simulink model "MATLABPSB_BASED_MODELING_AND_Sim"  (Simulink 8.1)
settings: Solver=FixedStepDiscrete  SolverMode=SingleTasking  StartTime=0.0  StopTime=1  FixedStep=Ts  MaxStep=Ts*2  RelTol=1e-4  AbsTol=1e-4
PreLoadFcn:
  | Ts=50e-6;
values from neighbouring files (symbols this model uses):
  A = 1.5    [LoadSimulation.m]
undefined symbols (not defined in the file or in its folder): DiscIntNeverNeededParam, find_system
libraries: powerlib x205, powerlib_extras x39
(part 2 of 5)

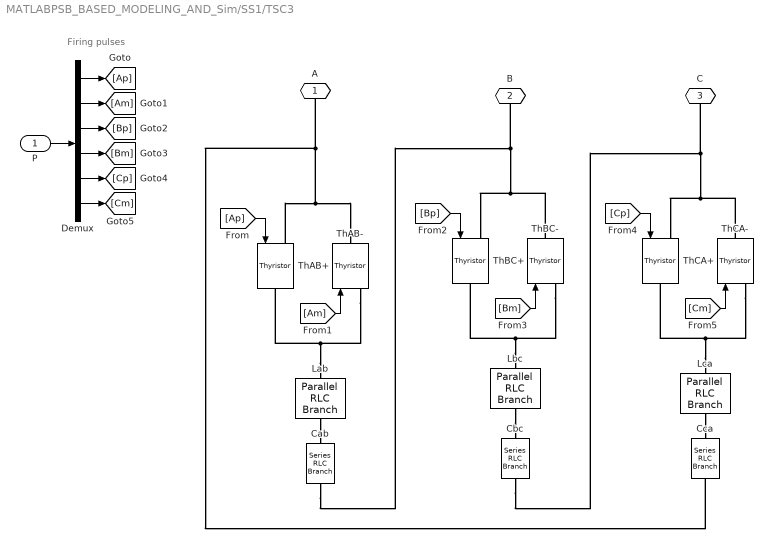
== system MATLABPSB_BASED_MODELING_AND_Sim/SS1/TSC3 ==
  note: Firing pulses
  P : Inport  PortDimensions=6
  Cab : powerlib/Elements/Series RLC Branch  LConnTagsString=__new0  RConnTagsString=__new0  BranchType=RC  Resistance=Rseries  Inductance=1.0  SetiL0=off  InitialCurrent=0  Capacitance=Ccmt  Setx0=off  InitialVoltage=0  Measurements=Branch voltage and current
  Cbc : powerlib/Elements/Series RLC Branch  LConnTagsString=__new0  RConnTagsString=__new0  BranchType=RC  Resistance=Rseries  Inductance=1.0  SetiL0=off  InitialCurrent=0  Capacitance=Ccmt  Setx0=off  InitialVoltage=0  Measurements=None
  Cca : powerlib/Elements/Series RLC Branch  LConnTagsString=__new0  RConnTagsString=__new0  BranchType=RC  Resistance=Rseries  Inductance=1.0  SetiL0=off  InitialCurrent=0  Capacitance=Ccmt  Setx0=off  InitialVoltage=0  Measurements=None
  Demux : Demux  Outputs=6
  Lab : powerlib/Elements/Parallel RLC Branch  LConnTagsString=a  RConnTagsString=__new0  BranchType=RL  Resistance=Rparallel  Inductance=Lcmt  SetiL0=off  InitialCurrent=0  Capacitance=1.0  Setx0=off  InitialVoltage=0  Measurements=None
  Lbc : powerlib/Elements/Parallel RLC Branch  LConnTagsString=a  RConnTagsString=__new0  BranchType=RL  Resistance=Rparallel  Inductance=Lcmt  SetiL0=off  InitialCurrent=0  Capacitance=1.0  Setx0=off  InitialVoltage=0  Measurements=None
  Lca : powerlib/Elements/Parallel RLC Branch  LConnTagsString=a  RConnTagsString=__new0  BranchType=RL  Resistance=Rparallel  Inductance=Lcmt  SetiL0=off  InitialCurrent=0  Capacitance=1.0  Setx0=off  InitialVoltage=0  Measurements=None
  ThAB+ : powerlib/Power Electronics/Thyristor  Ron=Ron  Lon=0  Vf=Vf  IC=0  Rs=Rsnub  Cs=Csnub  Measurements=off
      settings: AttributesFormatString=\n
  ThAB- : powerlib/Power Electronics/Thyristor  Ron=Ron  Lon=0  Vf=Vf  IC=0  Rs=inf  Cs=0  Measurements=off
      settings: AttributesFormatString=\n
  ThBC+ : powerlib/Power Electronics/Thyristor  Ron=Ron  Lon=0  Vf=Vf  IC=0  Rs=Rsnub  Cs=Csnub  Measurements=off
      settings: AttributesFormatString=\n
  ThBC- : powerlib/Power Electronics/Thyristor  Ron=Ron  Lon=0  Vf=Vf  IC=0  Rs=inf  Cs=0  Measurements=off
      settings: AttributesFormatString=\n
  ThCA+ : powerlib/Power Electronics/Thyristor  Ron=Ron  Lon=0  Vf=Vf  IC=0  Rs=Rsnub  Cs=Csnub  Measurements=off
      settings: AttributesFormatString=\n
  ThCA- : powerlib/Power Electronics/Thyristor  Ron=Ron  Lon=0  Vf=Vf  IC=0  Rs=inf  Cs=0  Measurements=off
      settings: AttributesFormatString=\n
  A : PMIOPort  Port=1  Side=Left
  B : PMIOPort  Port=2  Side=Left
  C : PMIOPort  Port=3  Side=Left
  wires:
  P/1 -> Demux/1
  [Ap] -> ThAB+/1
  Demux/1 -> [Ap]
  Demux/2 -> [Am]
  Demux/3 -> [Bp]
  Demux/4 -> [Bm]
  Demux/5 -> [Cp]
  [Am] -> ThAB-/1
  [Bp] -> ThBC+/1
  [Bm] -> ThBC-/1
  [Cp] -> ThCA+/1
  [Cm] -> ThCA-/1
  Demux/6 -> [Cm]
  connections:
  Lab/RConn1 -- Cab/LConn1
  Lab/LConn1 -- ThAB-/LConn1 -- ThAB+/RConn1
  Cca/RConn1 -- A/RConn1 -- ThAB+/LConn1 -- ThAB-/RConn1
  Lbc/LConn1 -- ThBC-/LConn1 -- ThBC+/RConn1
  Cab/RConn1 -- ThBC-/RConn1 -- ThBC+/LConn1 -- B/RConn1
  Lca/LConn1 -- ThCA-/LConn1 -- ThCA+/RConn1
  Cbc/RConn1 -- ThCA-/RConn1 -- ThCA+/LConn1 -- C/RConn1
  Lbc/RConn1 -- Cbc/LConn1
  Lca/RConn1 -- Cca/LConn1

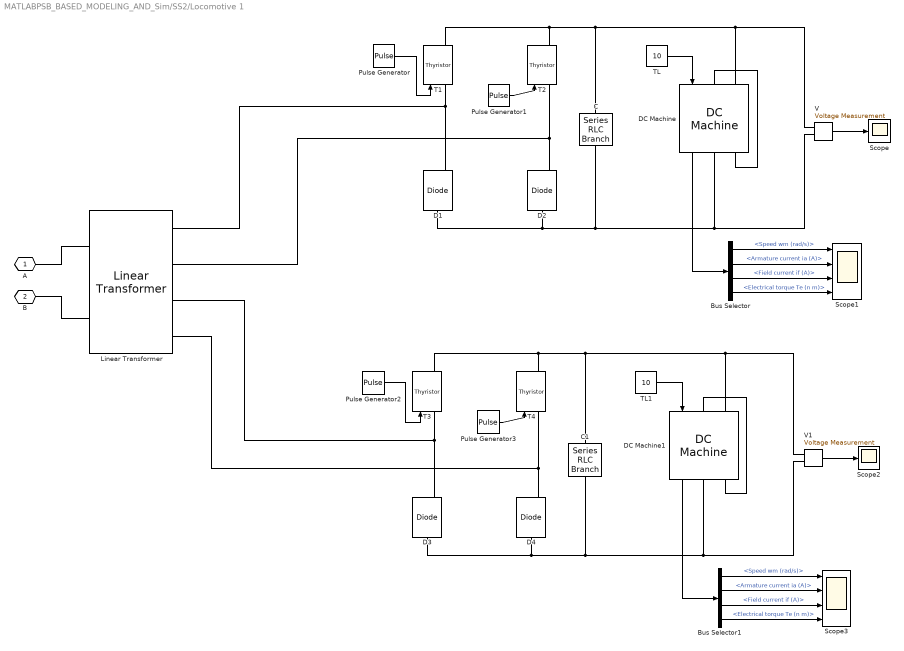
== system MATLABPSB_BASED_MODELING_AND_Sim/SS2/Locomotive 1 ==
  Bus Selector : BusSelector  OutputSignals=Speed wm (rad/s),Armature current ia (A),Field current if (A),Electrical torque Te (n m)
  Bus Selector1 : BusSelector  OutputSignals=Speed wm (rad/s),Armature current ia (A),Field current if (A),Electrical torque Te (n m)
  C : powerlib/Elements/Series RLC Branch  LConnTagsString=__new0  RConnTagsString=__new0  BranchType=C  Resistance=1000  Inductance=1e-3  SetiL0=off  InitialCurrent=0  Capacitance=2000e-6  Setx0=on  InitialVoltage=400  Measurements=None
  C1 : powerlib/Elements/Series RLC Branch  LConnTagsString=__new0  RConnTagsString=__new0  BranchType=C  Resistance=1000  Inductance=1e-3  SetiL0=off  InitialCurrent=0  Capacitance=2000e-6  Setx0=on  InitialVoltage=400  Measurements=None
  D{1..4} (4 alike) : powerlib/Power Electronics/Diode  Ron=0.001  Lon=0  Vf=0.8  IC=0  UseSnubber=off  Rs=500  Cs=250e-9  Measurements=on
  DC Machine : powerlib/Machines/DC Machine  PresetModel=No  MechanicalLoad=Torque TL  FieldType=Wound  ShowDetailedParameters=on  RLa="[ 2.6  150e-3]"  RLf=[0.6 20e-3]  Laf=1.8  MachineConstant=Torque constant (N.m/A)  Ke=1.8  Kt=1.8  J=0.1  Bm=0  Tf=0  w0=1  Ifinit=1  TsPowergui=0  TsBlock=-1
  DC Machine1 : powerlib/Machines/DC Machine  PresetModel=No  MechanicalLoad=Torque TL  FieldType=Wound  ShowDetailedParameters=on  RLa="[ 2.6  150e-3]"  RLf=[0.6 20e-3]  Laf=1.8  MachineConstant=Torque constant (N.m/A)  Ke=1.8  Kt=1.8  J=0.1  Bm=0  Tf=0  w0=1  Ifinit=1  TsPowergui=0  TsBlock=-1
  Linear Transformer : powerlib/Elements/Linear Transformer  LConnTagsString=a|b  RConnTagsString=A|B|C|D  UNITS=pu  NominalPower=[ 10e6 50 ]  winding1="[ 25e3  0.0001  0.04 ]"  winding2="[ 400  0.0001  0.02 ]"  ThreeWindings=on  winding3="[ 400  0.0001  0.02 ]"  RmLm=[ 500 500 ]  Measurements=None  DataType=off
  Pulse Generator : DiscretePulseGenerator  PulseType=Time based  Period=20e-3  PulseWidth=3
  Pulse Generator1 : DiscretePulseGenerator  PulseType=Time based  Period=20e-3  PulseWidth=3  PhaseDelay=10e-3
  Pulse Generator2 : DiscretePulseGenerator  PulseType=Time based  Period=20e-3  PulseWidth=3
  Pulse Generator3 : DiscretePulseGenerator  PulseType=Time based  Period=20e-3  PulseWidth=3  PhaseDelay=10e-3
  Scope : Scope
      settings: YMin=-50  YMax=800  SaveName=ScopeData3  Decimation=5
  Scope1 : Scope  NumInputPorts=4
      settings: YMin=0~-5~-5~-5  YMax=100~5~5~20  SaveName=ScopeData4  Decimation=5
  Scope2 : Scope
      settings: YMin=-50  YMax=800  SaveName=ScopeData5  Decimation=5
  Scope3 : Scope  NumInputPorts=4
      settings: YMin=0~-5~-5~-5  YMax=100~5~5~20  SaveName=ScopeData6  Decimation=5
  T{1..4} (4 alike) : powerlib/Power Electronics/Thyristor  Ron=0.001  Lon=0  Vf=0.8  IC=0  Rs=500  Cs=250e-9  Measurements=on
  TL : Constant  Value=10
  TL1 : Constant  Value=10
  V : powerlib/Measurements/Voltage Measurement  PhasorSimulation=off  OutputType=Complex  PSBequivalent=0
  V1 : powerlib/Measurements/Voltage Measurement  PhasorSimulation=off  OutputType=Complex  PSBequivalent=0
  A : PMIOPort  Tag=PMCPort  Port=1  Side=Left
  B : PMIOPort  Tag=PMCPort  Port=2  Side=Left
  wires:
  Pulse Generator/1 -> T1/1
  Pulse Generator1/1 -> T2/1
  V/1 -> Scope/1
  TL/1 -> DC Machine/1
  DC Machine/1 -> Bus Selector/1
  Bus Selector/1 -> Scope1/1  "<Speed wm (rad/s)>"
  Bus Selector/2 -> Scope1/2  "<Armature current ia (A)>"
  Bus Selector/3 -> Scope1/3  "<Field current if (A)>"
  Bus Selector/4 -> Scope1/4  "<Electrical torque Te (n m)>"
  Pulse Generator2/1 -> T3/1
  Pulse Generator3/1 -> T4/1
  V1/1 -> Scope2/1
  TL1/1 -> DC Machine1/1
  DC Machine1/1 -> Bus Selector1/1
  Bus Selector1/1 -> Scope3/1  "<Speed wm (rad/s)>"
  Bus Selector1/2 -> Scope3/2  "<Armature current ia (A)>"
  Bus Selector1/3 -> Scope3/3  "<Field current if (A)>"
  Bus Selector1/4 -> Scope3/4  "<Electrical torque Te (n m)>"
  connections:
  D1/RConn1 -- Linear Transformer/RConn1 -- T1/LConn1
  D2/RConn1 -- Linear Transformer/RConn2 -- T2/LConn1
  T1/RConn1 -- T2/RConn1 -- C/LConn1 -- V/LConn1 -- DC Machine/LConn2
  D1/LConn1 -- D2/LConn1 -- C/RConn1 -- V/LConn2 -- DC Machine/RConn1
  DC Machine/RConn2 -- DC Machine/LConn1
  T3/RConn1 -- T4/RConn1 -- V1/LConn1 -- DC Machine1/LConn2 -- C1/LConn1
  D3/LConn1 -- D4/LConn1 -- V1/LConn2 -- DC Machine1/RConn1 -- C1/RConn1
  DC Machine1/RConn2 -- DC Machine1/LConn1
  D4/RConn1 -- T4/LConn1 -- Linear Transformer/RConn4
  D3/RConn1 -- T3/LConn1 -- Linear Transformer/RConn3
  A/RConn1 -- Linear Transformer/LConn1
  B/RConn1 -- Linear Transformer/LConn2

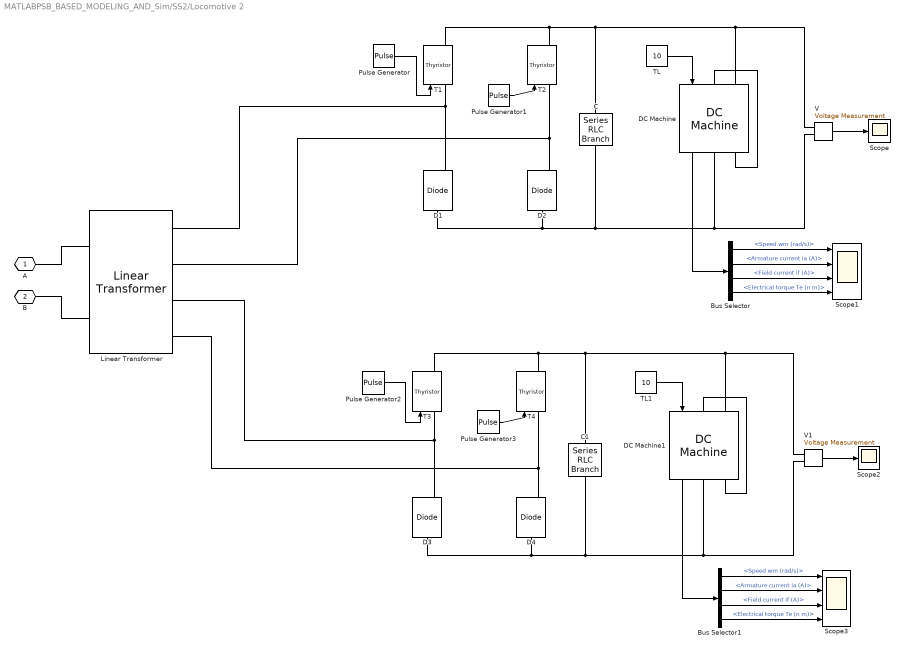
== system MATLABPSB_BASED_MODELING_AND_Sim/SS2/Locomotive 2 ==
  Bus Selector : BusSelector  OutputSignals=Speed wm (rad/s),Armature current ia (A),Field current if (A),Electrical torque Te (n m)
  Bus Selector1 : BusSelector  OutputSignals=Speed wm (rad/s),Armature current ia (A),Field current if (A),Electrical torque Te (n m)
  C : powerlib/Elements/Series RLC Branch  LConnTagsString=__new0  RConnTagsString=__new0  BranchType=C  Resistance=1000  Inductance=1e-3  SetiL0=off  InitialCurrent=0  Capacitance=2000e-6  Setx0=on  InitialVoltage=400  Measurements=None
  C1 : powerlib/Elements/Series RLC Branch  LConnTagsString=__new0  RConnTagsString=__new0  BranchType=C  Resistance=1000  Inductance=1e-3  SetiL0=off  InitialCurrent=0  Capacitance=2000e-6  Setx0=on  InitialVoltage=400  Measurements=None
  D{1..4} (4 alike) : powerlib/Power Electronics/Diode  Ron=0.001  Lon=0  Vf=0.8  IC=0  UseSnubber=off  Rs=500  Cs=250e-9  Measurements=on
  DC Machine : powerlib/Machines/DC Machine  PresetModel=No  MechanicalLoad=Torque TL  FieldType=Wound  ShowDetailedParameters=on  RLa="[ 2.6  150e-3]"  RLf=[0.6 20e-3]  Laf=1.8  MachineConstant=Torque constant (N.m/A)  Ke=1.8  Kt=1.8  J=0.1  Bm=0  Tf=0  w0=1  Ifinit=1  TsPowergui=0  TsBlock=-1
  DC Machine1 : powerlib/Machines/DC Machine  PresetModel=No  MechanicalLoad=Torque TL  FieldType=Wound  ShowDetailedParameters=on  RLa="[ 2.6  150e-3]"  RLf=[0.6 20e-3]  Laf=1.8  MachineConstant=Torque constant (N.m/A)  Ke=1.8  Kt=1.8  J=0.1  Bm=0  Tf=0  w0=1  Ifinit=1  TsPowergui=0  TsBlock=-1
  Linear Transformer : powerlib/Elements/Linear Transformer  LConnTagsString=a|b  RConnTagsString=A|B|C|D  UNITS=pu  NominalPower=[ 10e6 50 ]  winding1="[ 25e3  0.0001  0.04 ]"  winding2="[ 400  0.0001  0.02 ]"  ThreeWindings=on  winding3="[ 400  0.0001  0.02 ]"  RmLm=[ 500 500 ]  Measurements=None  DataType=off
  Pulse Generator : DiscretePulseGenerator  PulseType=Time based  Period=20e-3  PulseWidth=3
  Pulse Generator1 : DiscretePulseGenerator  PulseType=Time based  Period=20e-3  PulseWidth=3  PhaseDelay=10e-3
  Pulse Generator2 : DiscretePulseGenerator  PulseType=Time based  Period=20e-3  PulseWidth=3
  Pulse Generator3 : DiscretePulseGenerator  PulseType=Time based  Period=20e-3  PulseWidth=3  PhaseDelay=10e-3
  Scope : Scope
      settings: YMin=-50  YMax=800  SaveName=ScopeData3  Decimation=5
  Scope1 : Scope  NumInputPorts=4
      settings: YMin=0~-5~-5~-5  YMax=100~5~5~20  SaveName=ScopeData4  Decimation=5
  Scope2 : Scope
      settings: YMin=-50  YMax=800  SaveName=ScopeData5  Decimation=5
  Scope3 : Scope  NumInputPorts=4
      settings: YMin=0~-5~-5~-5  YMax=100~5~5~20  SaveName=ScopeData6  Decimation=5
  T{1..4} (4 alike) : powerlib/Power Electronics/Thyristor  Ron=0.001  Lon=0  Vf=0.8  IC=0  Rs=500  Cs=250e-9  Measurements=on
  TL : Constant  Value=10
  TL1 : Constant  Value=10
  V : powerlib/Measurements/Voltage Measurement  PhasorSimulation=off  OutputType=Complex  PSBequivalent=0
  V1 : powerlib/Measurements/Voltage Measurement  PhasorSimulation=off  OutputType=Complex  PSBequivalent=0
  A : PMIOPort  Tag=PMCPort  Port=1  Side=Left
  B : PMIOPort  Tag=PMCPort  Port=2  Side=Left
  wires:
  Pulse Generator/1 -> T1/1
  Pulse Generator1/1 -> T2/1
  V/1 -> Scope/1
  TL/1 -> DC Machine/1
  DC Machine/1 -> Bus Selector/1
  Bus Selector/1 -> Scope1/1  "<Speed wm (rad/s)>"
  Bus Selector/2 -> Scope1/2  "<Armature current ia (A)>"
  Bus Selector/3 -> Scope1/3  "<Field current if (A)>"
  Bus Selector/4 -> Scope1/4  "<Electrical torque Te (n m)>"
  Pulse Generator2/1 -> T3/1
  Pulse Generator3/1 -> T4/1
  V1/1 -> Scope2/1
  TL1/1 -> DC Machine1/1
  DC Machine1/1 -> Bus Selector1/1
  Bus Selector1/1 -> Scope3/1  "<Speed wm (rad/s)>"
  Bus Selector1/2 -> Scope3/2  "<Armature current ia (A)>"
  Bus Selector1/3 -> Scope3/3  "<Field current if (A)>"
  Bus Selector1/4 -> Scope3/4  "<Electrical torque Te (n m)>"
  connections:
  D1/RConn1 -- Linear Transformer/RConn1 -- T1/LConn1
  D2/RConn1 -- Linear Transformer/RConn2 -- T2/LConn1
  T1/RConn1 -- T2/RConn1 -- C/LConn1 -- V/LConn1 -- DC Machine/LConn2
  D1/LConn1 -- D2/LConn1 -- C/RConn1 -- V/LConn2 -- DC Machine/RConn1
  DC Machine/RConn2 -- DC Machine/LConn1
  T3/RConn1 -- T4/RConn1 -- V1/LConn1 -- DC Machine1/LConn2 -- C1/LConn1
  D3/LConn1 -- D4/LConn1 -- V1/LConn2 -- DC Machine1/RConn1 -- C1/RConn1
  DC Machine1/RConn2 -- DC Machine1/LConn1
  D4/RConn1 -- T4/LConn1 -- Linear Transformer/RConn4
  D3/RConn1 -- T3/LConn1 -- Linear Transformer/RConn3
  A/RConn1 -- Linear Transformer/LConn1
  B/RConn1 -- Linear Transformer/LConn2

== system MATLABPSB_BASED_MODELING_AND_Sim/SS2/SVC Controller ==
  note: Pulses
  note: SVC Controller
  note: Pierre Giroux, Gilbert Sybille
      | Power System Laboratory, IREQ
      | Hydro-Quebec
  note: used for misfiring
      | simulation
  Vabc_prim : Inport  PortDimensions=3
  Vabc_sec : Inport  Port=2  PortDimensions=3
  3-phase signal generator : Subsystem
  Constant : Constant  Value=0.00000001
  Constant1 : Constant  Value=Bref
  Demux : Demux  Outputs=[1 5]
  Distribution Unit : Subsystem  mask(Distribution Unit){ParNom=[333e6 60], Xf_xfo=0.15, Vsec_svc=16e3, L_TCR=18.7e-3, C_TSC=308.4e-6, L_TSC=1.13e-3, hyst_svc=0.1, Ts=Ts}
      mask prompts: ParNom "Transformer nominal power and frequency: [  P (VA)    Freq (Hz)  ]"; Xf_xfo "Transformer total leakage (pu/Pnom):"; Vsec_svc "Nominal secondary voltage (Volts rms ph-ph):"; L_TCR "TCR branch inductance (H):"; C_TSC "TSC branch capacitance (F):"; L_TSC "TSC branch inductance (H)"; hyst_svc "Hysteresis - Distribution unit (pu/100MVA):"; Ts "Sample time:"
      mask init: same as MATLABPSB_BASED_MODELING_AND_Sim/SS1/SVC Controller/Distribution Unit
  Firing Unit : Subsystem  mask(Firing Unit){FiringMode=Synchronized, Nstep=0, ParInit=[0 60], Ts=Ts}
      mask prompts: FiringMode "Firing mode"; Nstep "Total delay (in number of time step)"; ParInit "Initial phase and frequency of input: [ Phase (degree)  Freq (Hz) ]"; Ts "Sample time:"
      mask init:
      | PhaseInit=ParInit(1);
      | FreqInit=ParInit(2);
      mask TypeOptions FiringMode: Synchronized | Continuous
  Logical Operator : Logic  Operator=OR
  Manual  Switch : ManualSwitch
  Measurement System : Subsystem  mask(SVC measurement system){Vnom=735e3, ParI=[735e3*0.9998 0 60], Ts=Ts}
      mask prompts: Vnom "Nominal voltage (volts rms ph-ph)"; ParI "Initial input: [ Mag (volts rms ph-ph)  Phase (degree) Freq (Hz) ]"; Ts "Sample time:"
      mask init:
      | Mag_Init=ParI(1)/Vnom;
      | Phase_Init=ParI(2);
      | Freq_Init=ParI(3);
  Mux2 : Mux  Inputs=[1 5]
  Sum : Sum  Inputs=|++  SaturateOnIntegerOverflow=on
  Timer : powerlib_extras/Control  Blocks/Timer  t="[ 0  0.121  0.121+eps ]*100"  e="[0  1  0 ]"
  Timer2 : powerlib_extras/Control  Blocks/Timer  t="[ 0  0.4  0.6 ]"  e=[1 1 1 ]
  Voltage Regulator : Subsystem
  TCR : Outport
  TSC1 : Outport  Port=2
  TSC2 : Outport  Port=3
  TSC3 : Outport  Port=4
  wires:
  Timer/1 -> Logical Operator/1
  Firing Unit/2(TSC1_Pulses) -> Demux/1
  Measurement System/1(Vmes) -> Voltage Regulator/1(Vmes)
  Constant1/1 -> Voltage Regulator/2(Bref)
  Mux2/1 -> TSC1/1
  Demux/2 -> Mux2/2
  Logical Operator/1 -> Mux2/1
  Demux/1 -> Logical Operator/2
  Voltage Regulator/1(Bsvc) -> Distribution Unit/1(Bsvc)
  Sum/1 -> Voltage Regulator/3(Vref)
  Constant/1 -> Sum/1
  Timer2/1 -> Sum/2
  Vabc_prim/1 -> Manual  Switch/1
  Manual  Switch/1 -> Measurement System/1(Vabc)
  3-phase signal generator/1(abc) -> Manual  Switch/2
  Firing Unit/1(TCR_Pulses) -> TCR/1
  Firing Unit/3(TSC2_Pulses) -> TSC2/1
  Firing Unit/4(TSC3_Pulses) -> TSC3/1
  Distribution Unit/1(Alpha) -> Firing Unit/2(Alpha)
  Distribution Unit/2(TSC1_On) -> Firing Unit/3(TSC1_On)
  Distribution Unit/3(TSC2_On) -> Firing Unit/4(TSC2_On)
  Distribution Unit/4(TSC3_On) -> Firing Unit/5(TSC3_On)
  Vabc_sec/1 -> Firing Unit/1(Vabc)

== system MATLABPSB_BASED_MODELING_AND_Sim/SS2/TCR ==
  note: Firing pulses
  note: TCR
  P : Inport  PortDimensions=6
  Demux : Demux  Outputs=6
  Lab : powerlib/Elements/Series RLC Branch  LConnTagsString=__new0  RConnTagsString=__new0  BranchType=RL  Resistance=Rtcr  Inductance=Ltcr  SetiL0=off  InitialCurrent=0  Capacitance=1.0  Setx0=off  InitialVoltage=0  Measurements=Branch current
  Lbc : powerlib/Elements/Series RLC Branch  LConnTagsString=__new0  RConnTagsString=__new0  BranchType=RL  Resistance=Rtcr  Inductance=Ltcr  SetiL0=off  InitialCurrent=0  Capacitance=1.0  Setx0=off  InitialVoltage=0  Measurements=None
  Lca : powerlib/Elements/Series RLC Branch  LConnTagsString=__new0  RConnTagsString=__new0  BranchType=RL  Resistance=Rtcr  Inductance=Ltcr  SetiL0=off  InitialCurrent=0  Capacitance=1.0  Setx0=off  InitialVoltage=0  Measurements=None
  ThAB+ : powerlib/Power Electronics/Thyristor  Ron=Ron  Lon=0  Vf=Vf  IC=0  Rs=Rsnub  Cs=Csnub  Measurements=off
      settings: AttributesFormatString=\n
  ThAB- : powerlib/Power Electronics/Thyristor  Ron=Ron  Lon=0  Vf=Vf  IC=0  Rs=inf  Cs=0  Measurements=off
      settings: AttributesFormatString=\n
  ThBC+ : powerlib/Power Electronics/Thyristor  Ron=Ron  Lon=0  Vf=Vf  IC=0  Rs=Rsnub  Cs=Csnub  Measurements=off
      settings: AttributesFormatString=\n
  ThBC- : powerlib/Power Electronics/Thyristor  Ron=Ron  Lon=0  Vf=Vf  IC=0  Rs=inf  Cs=0  Measurements=off
      settings: AttributesFormatString=\n
  ThCA+ : powerlib/Power Electronics/Thyristor  Ron=Ron  Lon=0  Vf=Vf  IC=0  Rs=Rsnub  Cs=Csnub  Measurements=off
      settings: AttributesFormatString=\n
  ThCA- : powerlib/Power Electronics/Thyristor  Ron=Ron  Lon=0  Vf=Vf  IC=0  Rs=inf  Cs=0  Measurements=off
      settings: AttributesFormatString=\n
  A : PMIOPort  Port=1  Side=Left
  B : PMIOPort  Port=2  Side=Left
  C : PMIOPort  Port=3  Side=Left
  wires:
  P/1 -> Demux/1
  Demux/1 -> [Ap]
  Demux/2 -> [Am]
  Demux/3 -> [Bp]
  Demux/4 -> [Bm]
  Demux/5 -> [Cp]
  [Cp] -> ThCA+/1
  [Cm] -> ThCA-/1
  Demux/6 -> [Cm]
  [Bm] -> ThBC-/1
  [Bp] -> ThBC+/1
  [Am] -> ThAB-/1
  [Ap] -> ThAB+/1
  connections:
  ThAB-/LConn1 -- ThAB+/RConn1 -- Lab/LConn1
  ThAB+/LConn1 -- ThAB-/RConn1 -- Lca/RConn1 -- A/RConn1
  ThBC-/LConn1 -- Lbc/LConn1 -- ThBC+/RConn1
  Lab/RConn1 -- ThBC-/RConn1 -- ThBC+/LConn1 -- B/RConn1
  Lca/LConn1 -- ThCA-/LConn1 -- ThCA+/RConn1
  Lbc/RConn1 -- ThCA-/RConn1 -- ThCA+/LConn1 -- C/RConn1

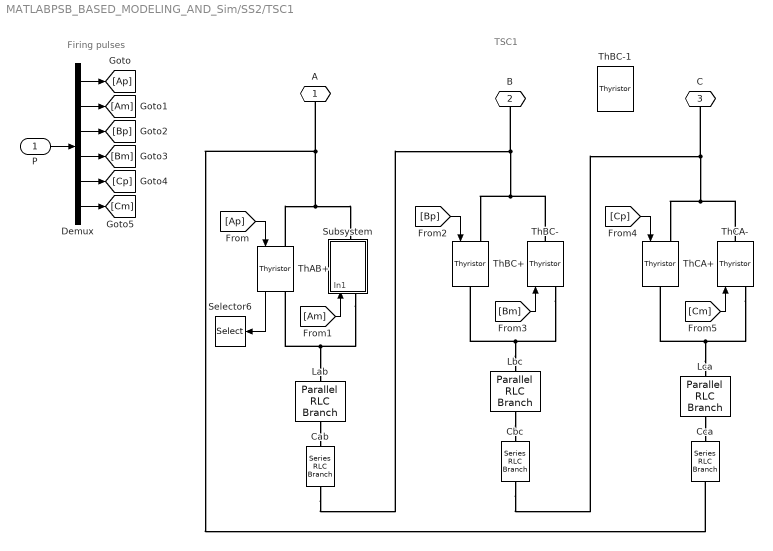
== system MATLABPSB_BASED_MODELING_AND_Sim/SS2/TSC1 ==
  note: Firing pulses
  note: TSC1
  P : Inport  PortDimensions=6
  Cab : powerlib/Elements/Series RLC Branch  LConnTagsString=__new0  RConnTagsString=__new0  BranchType=RC  Resistance=Rseries  Inductance=1.0  SetiL0=off  InitialCurrent=0  Capacitance=Ccmt  Setx0=off  InitialVoltage=0  Measurements=Branch voltage and current
  Cbc : powerlib/Elements/Series RLC Branch  LConnTagsString=__new0  RConnTagsString=__new0  BranchType=RC  Resistance=Rseries  Inductance=1.0  SetiL0=off  InitialCurrent=0  Capacitance=Ccmt  Setx0=off  InitialVoltage=0  Measurements=None
  Cca : powerlib/Elements/Series RLC Branch  LConnTagsString=__new0  RConnTagsString=__new0  BranchType=RC  Resistance=Rseries  Inductance=1.0  SetiL0=off  InitialCurrent=0  Capacitance=Ccmt  Setx0=off  InitialVoltage=0  Measurements=None
  Demux : Demux  Outputs=6
  Lab : powerlib/Elements/Parallel RLC Branch  LConnTagsString=a  RConnTagsString=__new0  BranchType=RL  Resistance=Rparallel  Inductance=Lcmt  SetiL0=off  InitialCurrent=0  Capacitance=1.0  Setx0=off  InitialVoltage=0  Measurements=None
  Lbc : powerlib/Elements/Parallel RLC Branch  LConnTagsString=a  RConnTagsString=__new0  BranchType=RL  Resistance=Rparallel  Inductance=Lcmt  SetiL0=off  InitialCurrent=0  Capacitance=1.0  Setx0=off  InitialVoltage=0  Measurements=None
  Lca : powerlib/Elements/Parallel RLC Branch  LConnTagsString=a  RConnTagsString=__new0  BranchType=RL  Resistance=Rparallel  Inductance=Lcmt  SetiL0=off  InitialCurrent=0  Capacitance=1.0  Setx0=off  InitialVoltage=0  Measurements=None
  Selector6 : Selector  InputPortWidth=2  IndexOptions=Index vector (dialog)  Indices=2  OutputSizes=1
  Subsystem : Subsystem  mask(Thyristor){Ron=Ron, Lon=0, Vf=Vf, IC=0, Rs=inf, Cs=0, Measurements=off}
      mask prompts: Ron "Resistance Ron (Ohms) :"; Lon "Inductance Lon (H) :"; Vf "Forward voltage Vf (V) :"; IC "Initial current Ic (A) :"; Rs "Snubber resistance Rs (Ohms) :"; Cs "Snubber capacitance Cs (F) :"; Measurements "Show measurement port"
      mask help:
      | Thyristor in parallel with a series RC snubber circuit.
      | In on-state the Thyristor model has an internal resistance (Ron) and inductance (Lon).
      | For most applications the internal inductance should be set to zero.
      | In off-state the Thyristor as an infinite impedance.
      mask Help: helpview(psbhelp);
      mask TypeOptions Ron: ThAB-/Ron
      mask TypeOptions Lon: ThAB-/Lon
      mask TypeOptions Vf: ThAB-/Vf
      mask TypeOptions IC: ThAB-/IC
      mask TypeOptions Rs: ThAB-/Rs
      mask TypeOptions Cs: ThAB-/Cs
      mask TypeOptions Measurements: ThAB-/Measurements
  ThAB+ : powerlib/Power Electronics/Thyristor  Ron=Ron  Lon=0  Vf=Vf  IC=0  Rs=Rsnub  Cs=Csnub  Measurements=on
      settings: AttributesFormatString=\n
  ThBC+ : powerlib/Power Electronics/Thyristor  Ron=Ron  Lon=0  Vf=Vf  IC=0  Rs=Rsnub  Cs=Csnub  Measurements=off
      settings: AttributesFormatString=\n
  ThBC- : powerlib/Power Electronics/Thyristor  Ron=Ron  Lon=0  Vf=Vf  IC=0  Rs=inf  Cs=0  Measurements=off
      settings: AttributesFormatString=\n
  ThBC-1 : powerlib/Power Electronics/Thyristor  Ron=Ron  Lon=0  Vf=Vf  IC=0  Rs=inf  Cs=0  Measurements=off
      settings: AttributesFormatString=\n
  ThCA+ : powerlib/Power Electronics/Thyristor  Ron=Ron  Lon=0  Vf=Vf  IC=0  Rs=Rsnub  Cs=Csnub  Measurements=off
      settings: AttributesFormatString=\n
  ThCA- : powerlib/Power Electronics/Thyristor  Ron=Ron  Lon=0  Vf=Vf  IC=0  Rs=inf  Cs=0  Measurements=off
      settings: AttributesFormatString=\n
  A : PMIOPort  Port=1  Side=Left
  B : PMIOPort  Port=2  Side=Left
  C : PMIOPort  Port=3  Side=Left
  wires:
  P/1 -> Demux/1
  [Ap] -> ThAB+/1
  Demux/1 -> [Ap]
  Demux/2 -> [Am]
  Demux/3 -> [Bp]
  Demux/4 -> [Bm]
  Demux/5 -> [Cp]
  [Am] -> Subsystem/1(In1)
  [Bp] -> ThBC+/1
  [Bm] -> ThBC-/1
  [Cp] -> ThCA+/1
  [Cm] -> ThCA-/1
  Demux/6 -> [Cm]
  ThAB+/1 -> Selector6/1
  connections:
  Lab/RConn1 -- Cab/LConn1
  ThAB+/RConn1 -- Subsystem/LConn1 -- Lab/LConn1
  Cca/RConn1 -- A/RConn1 -- ThAB+/LConn1 -- Subsystem/RConn1
  Lbc/LConn1 -- ThBC-/LConn1 -- ThBC+/RConn1
  Cab/RConn1 -- ThBC-/RConn1 -- ThBC+/LConn1 -- B/RConn1
  Lca/LConn1 -- ThCA-/LConn1 -- ThCA+/RConn1
  Cbc/RConn1 -- ThCA-/RConn1 -- ThCA+/LConn1 -- C/RConn1
  Lbc/RConn1 -- Cbc/LConn1
  Lca/RConn1 -- Cca/LConn1

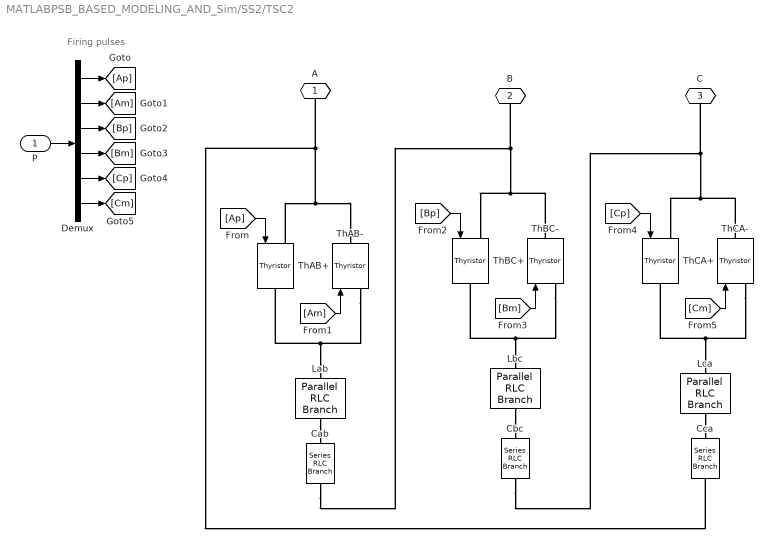
== system MATLABPSB_BASED_MODELING_AND_Sim/SS2/TSC2 ==
  note: Firing pulses
  P : Inport  PortDimensions=6
  Cab : powerlib/Elements/Series RLC Branch  LConnTagsString=__new0  RConnTagsString=__new0  BranchType=RC  Resistance=Rseries  Inductance=1.0  SetiL0=off  InitialCurrent=0  Capacitance=Ccmt  Setx0=off  InitialVoltage=0  Measurements=Branch voltage and current
  Cbc : powerlib/Elements/Series RLC Branch  LConnTagsString=__new0  RConnTagsString=__new0  BranchType=RC  Resistance=Rseries  Inductance=1.0  SetiL0=off  InitialCurrent=0  Capacitance=Ccmt  Setx0=off  InitialVoltage=0  Measurements=None
  Cca : powerlib/Elements/Series RLC Branch  LConnTagsString=__new0  RConnTagsString=__new0  BranchType=RC  Resistance=Rseries  Inductance=1.0  SetiL0=off  InitialCurrent=0  Capacitance=Ccmt  Setx0=off  InitialVoltage=0  Measurements=None
  Demux : Demux  Outputs=6
  Lab : powerlib/Elements/Parallel RLC Branch  LConnTagsString=a  RConnTagsString=__new0  BranchType=RL  Resistance=Rparallel  Inductance=Lcmt  SetiL0=off  InitialCurrent=0  Capacitance=1.0  Setx0=off  InitialVoltage=0  Measurements=None
  Lbc : powerlib/Elements/Parallel RLC Branch  LConnTagsString=a  RConnTagsString=__new0  BranchType=RL  Resistance=Rparallel  Inductance=Lcmt  SetiL0=off  InitialCurrent=0  Capacitance=1.0  Setx0=off  InitialVoltage=0  Measurements=None
  Lca : powerlib/Elements/Parallel RLC Branch  LConnTagsString=a  RConnTagsString=__new0  BranchType=RL  Resistance=Rparallel  Inductance=Lcmt  SetiL0=off  InitialCurrent=0  Capacitance=1.0  Setx0=off  InitialVoltage=0  Measurements=None
  ThAB+ : powerlib/Power Electronics/Thyristor  Ron=Ron  Lon=0  Vf=Vf  IC=0  Rs=Rsnub  Cs=Csnub  Measurements=off
      settings: AttributesFormatString=\n
  ThAB- : powerlib/Power Electronics/Thyristor  Ron=Ron  Lon=0  Vf=Vf  IC=0  Rs=inf  Cs=0  Measurements=off
      settings: AttributesFormatString=\n
  ThBC+ : powerlib/Power Electronics/Thyristor  Ron=Ron  Lon=0  Vf=Vf  IC=0  Rs=Rsnub  Cs=Csnub  Measurements=off
      settings: AttributesFormatString=\n
  ThBC- : powerlib/Power Electronics/Thyristor  Ron=Ron  Lon=0  Vf=Vf  IC=0  Rs=inf  Cs=0  Measurements=off
      settings: AttributesFormatString=\n
  ThCA+ : powerlib/Power Electronics/Thyristor  Ron=Ron  Lon=0  Vf=Vf  IC=0  Rs=Rsnub  Cs=Csnub  Measurements=off
      settings: AttributesFormatString=\n
  ThCA- : powerlib/Power Electronics/Thyristor  Ron=Ron  Lon=0  Vf=Vf  IC=0  Rs=inf  Cs=0  Measurements=off
      settings: AttributesFormatString=\n
  A : PMIOPort  Port=1  Side=Left
  B : PMIOPort  Port=2  Side=Left
  C : PMIOPort  Port=3  Side=Left
  wires:
  Demux/6 -> [Cm]
  [Cm] -> ThCA-/1
  [Cp] -> ThCA+/1
  [Bm] -> ThBC-/1
  [Bp] -> ThBC+/1
  [Am] -> ThAB-/1
  Demux/5 -> [Cp]
  Demux/4 -> [Bm]
  Demux/3 -> [Bp]
  Demux/2 -> [Am]
  Demux/1 -> [Ap]
  [Ap] -> ThAB+/1
  P/1 -> Demux/1
  connections:
  Lca/RConn1 -- Cca/LConn1
  Lbc/RConn1 -- Cbc/LConn1
  C/RConn1 -- ThCA+/LConn1 -- ThCA-/RConn1 -- Cbc/RConn1
  ThCA+/RConn1 -- ThCA-/LConn1 -- Lca/LConn1
  B/RConn1 -- ThBC+/LConn1 -- ThBC-/RConn1 -- Cab/RConn1
  ThBC+/RConn1 -- ThBC-/LConn1 -- Lbc/LConn1
  ThAB-/RConn1 -- ThAB+/LConn1 -- A/RConn1 -- Cca/RConn1
  ThAB+/RConn1 -- ThAB-/LConn1 -- Lab/LConn1
  Lab/RConn1 -- Cab/LConn1

== system MATLABPSB_BASED_MODELING_AND_Sim/SS2/TSC3 ==
  note: Firing pulses
  P : Inport  PortDimensions=6
  Cab : powerlib/Elements/Series RLC Branch  LConnTagsString=__new0  RConnTagsString=__new0  BranchType=RC  Resistance=Rseries  Inductance=1.0  SetiL0=off  InitialCurrent=0  Capacitance=Ccmt  Setx0=off  InitialVoltage=0  Measurements=Branch voltage and current
  Cbc : powerlib/Elements/Series RLC Branch  LConnTagsString=__new0  RConnTagsString=__new0  BranchType=RC  Resistance=Rseries  Inductance=1.0  SetiL0=off  InitialCurrent=0  Capacitance=Ccmt  Setx0=off  InitialVoltage=0  Measurements=None
  Cca : powerlib/Elements/Series RLC Branch  LConnTagsString=__new0  RConnTagsString=__new0  BranchType=RC  Resistance=Rseries  Inductance=1.0  SetiL0=off  InitialCurrent=0  Capacitance=Ccmt  Setx0=off  InitialVoltage=0  Measurements=None
  Demux : Demux  Outputs=6
  Lab : powerlib/Elements/Parallel RLC Branch  LConnTagsString=a  RConnTagsString=__new0  BranchType=RL  Resistance=Rparallel  Inductance=Lcmt  SetiL0=off  InitialCurrent=0  Capacitance=1.0  Setx0=off  InitialVoltage=0  Measurements=None
  Lbc : powerlib/Elements/Parallel RLC Branch  LConnTagsString=a  RConnTagsString=__new0  BranchType=RL  Resistance=Rparallel  Inductance=Lcmt  SetiL0=off  InitialCurrent=0  Capacitance=1.0  Setx0=off  InitialVoltage=0  Measurements=None
  Lca : powerlib/Elements/Parallel RLC Branch  LConnTagsString=a  RConnTagsString=__new0  BranchType=RL  Resistance=Rparallel  Inductance=Lcmt  SetiL0=off  InitialCurrent=0  Capacitance=1.0  Setx0=off  InitialVoltage=0  Measurements=None
  ThAB+ : powerlib/Power Electronics/Thyristor  Ron=Ron  Lon=0  Vf=Vf  IC=0  Rs=Rsnub  Cs=Csnub  Measurements=off
      settings: AttributesFormatString=\n
  ThAB- : powerlib/Power Electronics/Thyristor  Ron=Ron  Lon=0  Vf=Vf  IC=0  Rs=inf  Cs=0  Measurements=off
      settings: AttributesFormatString=\n
  ThBC+ : powerlib/Power Electronics/Thyristor  Ron=Ron  Lon=0  Vf=Vf  IC=0  Rs=Rsnub  Cs=Csnub  Measurements=off
      settings: AttributesFormatString=\n
  ThBC- : powerlib/Power Electronics/Thyristor  Ron=Ron  Lon=0  Vf=Vf  IC=0  Rs=inf  Cs=0  Measurements=off
      settings: AttributesFormatString=\n
  ThCA+ : powerlib/Power Electronics/Thyristor  Ron=Ron  Lon=0  Vf=Vf  IC=0  Rs=Rsnub  Cs=Csnub  Measurements=off
      settings: AttributesFormatString=\n
  ThCA- : powerlib/Power Electronics/Thyristor  Ron=Ron  Lon=0  Vf=Vf  IC=0  Rs=inf  Cs=0  Measurements=off
      settings: AttributesFormatString=\n
  A : PMIOPort  Port=1  Side=Left
  B : PMIOPort  Port=2  Side=Left
  C : PMIOPort  Port=3  Side=Left
  wires:
  P/1 -> Demux/1
  [Ap] -> ThAB+/1
  Demux/1 -> [Ap]
  Demux/2 -> [Am]
  Demux/3 -> [Bp]
  Demux/4 -> [Bm]
  Demux/5 -> [Cp]
  [Am] -> ThAB-/1
  [Bp] -> ThBC+/1
  [Bm] -> ThBC-/1
  [Cp] -> ThCA+/1
  [Cm] -> ThCA-/1
  Demux/6 -> [Cm]
  connections:
  Lab/RConn1 -- Cab/LConn1
  Lab/LConn1 -- ThAB-/LConn1 -- ThAB+/RConn1
  Cca/RConn1 -- A/RConn1 -- ThAB+/LConn1 -- ThAB-/RConn1
  Lbc/LConn1 -- ThBC-/LConn1 -- ThBC+/RConn1
  Cab/RConn1 -- ThBC-/RConn1 -- ThBC+/LConn1 -- B/RConn1
  Lca/LConn1 -- ThCA-/LConn1 -- ThCA+/RConn1
  Cbc/RConn1 -- ThCA-/RConn1 -- ThCA+/LConn1 -- C/RConn1
  Lbc/RConn1 -- Cbc/LConn1
  Lca/RConn1 -- Cca/LConn1

== system MATLABPSB_BASED_MODELING_AND_Sim/SS1/SVC Controller/3-phase signal generator ==
  Constant : Constant  Value=[0 -2*pi/3 2*pi/3]-2*pi/180
  Gain : Gain  Gain=2*pi*60  SaturateOnIntegerOverflow=on  OutDataTypeStr=Inherit: Same as input  ParamDataTypeStr=Inherit: Same as input
  Gain1 : Gain  Gain=0.9998  SaturateOnIntegerOverflow=on  OutDataTypeStr=Inherit: Same as input  ParamDataTypeStr=Inherit: Same as input
  Sum : Sum  Inputs=|++  SaturateOnIntegerOverflow=on
  Trigonometric Function : Trigonometry
  t : DigitalClock  SampleTime=Ts
  abc : Outport
  wires:
  Constant/1 -> Sum/2
  Sum/1 -> Trigonometric Function/1
  Trigonometric Function/1 -> Gain1/1
  t/1 -> Gain/1
  Gain/1 -> Sum/1
  Gain1/1 -> abc/1

== system MATLABPSB_BASED_MODELING_AND_Sim/SS1/SVC Controller/Distribution Unit ==
  note: Bsec = ( 2 - Alpha/90 + sin(2*Alpha)/PI ) * Bsec_nom
  Bsvc : Inport  PortDimensions=1
  Bprim-->Bsec : Fcn  Expr=u[1]/(1 + u[1]*Xf_xfo*100e6/Pnom_xfo)
  Bsec --> Alpha : Lookup  InputValues=B  Table=A  SaturateOnIntegerOverflow=on
  Saturation : Saturate  UpperLimit=0  LowerLimit=Bpu_TCR
  Sum1 : Sum  Inputs=+---  SaturateOnIntegerOverflow=on  InputSameDT=on  OutDataTypeStr=Inherit: Same as first input
  TSC1 : Relay  OnSwitchValue=0  OffSwitchValue=-1 * hyst_svc
  TSC1+TSC2 : Relay  OnSwitchValue=0+ Bpu_TSC  OffSwitchValue=-1 * hyst_svc + Bpu_TSC
  TSC1+TSC2+TSC3 : Relay  OnSwitchValue=0+ 2*Bpu_TSC  OffSwitchValue=-1 * hyst_svc + 2*Bpu_TSC
  pu100_puLnom : Gain  Gain=-1/Bpu_TCR  SaturateOnIntegerOverflow=on  OutDataTypeStr=Inherit: Same as input  ParamDataTypeStr=Inherit: Same as input
  pu100_puLnom1 : Gain  Gain=Bpu_TSC  SaturateOnIntegerOverflow=on  OutDataTypeStr=Inherit: Same as input  ParamDataTypeStr=Inherit: Same as input
  pu100_puLnom2 : Gain  Gain=Bpu_TSC  SaturateOnIntegerOverflow=on  OutDataTypeStr=Inherit: Same as input  ParamDataTypeStr=Inherit: Same as input
  pu100_puLnom3 : Gain  Gain=Bpu_TSC  SaturateOnIntegerOverflow=on  OutDataTypeStr=Inherit: Same as input  ParamDataTypeStr=Inherit: Same as input
  Alpha : Outport  InitialOutput=0
  TSC1_On : Outport  Port=2  InitialOutput=0
  TSC2_On : Outport  Port=3  InitialOutput=0
  TSC3_On : Outport  Port=4  InitialOutput=0
  wires:
  pu100_puLnom/1 -> Bsec --> Alpha/1
  Bsec --> Alpha/1 -> Alpha/1
  Bsvc/1 -> Bprim-->Bsec/1
  Bprim-->Bsec/1 -> TSC1/1, TSC1+TSC2/1, TSC1+TSC2+TSC3/1, Sum1/1
  Saturation/1 -> pu100_puLnom/1
  Sum1/1 -> Saturation/1
  pu100_puLnom2/1 -> Sum1/3
  pu100_puLnom3/1 -> Sum1/2
  TSC1/1 -> pu100_puLnom3/1, TSC1_On/1
  TSC1+TSC2/1 -> pu100_puLnom2/1, TSC2_On/1
  pu100_puLnom1/1 -> Sum1/4
  TSC1+TSC2+TSC3/1 -> pu100_puLnom1/1, TSC3_On/1

== system MATLABPSB_BASED_MODELING_AND_Sim/SS1/SVC Controller/Firing Unit ==
  Vabc : Inport  PortDimensions=3
  Alpha : Inport  Port=2  PortDimensions=1
  TSC1_On : Inport  Port=3  PortDimensions=1
  TSC2_On : Inport  Port=4  PortDimensions=1
  TSC3_On : Inport  Port=5  PortDimensions=1
  Demux : Demux  Outputs=3
  Firing Unit AB : Subsystem  mask{FiringMode=FiringMode, Nstep=Nstep, ParInit=[PhaseInit FreqInit], Ts=Ts}
      mask prompts: FiringMode "Firing Mode (1=Synchronized, 2=Continuous)"; Nstep "Total delay (in number of time step)"; ParInit "Initial phase and frequency of input: [ Phase (degree)  Freq (Hz) ]"; Ts "Sample time:"
      mask init:
      | PhaseInit=ParInit(1);
      | FreqInit=ParInit(2);
  Firing Unit BC : Subsystem  mask{FiringMode=FiringMode, Nstep=Nstep, ParInit=[PhaseInit-120 FreqInit], Ts=Ts}
      mask prompts: FiringMode "Firing Mode (1=Synchronized, 2=Continuous)"; Nstep "Total delay (in number of time step)"; ParInit "Initial phase and frequency of input: [ Phase (degree)  Freq (Hz) ]"; Ts "Sample time:"
      mask init:
      | PhaseInit=ParInit(1);
      | FreqInit=ParInit(2);
  Firing Unit CA : Subsystem  mask{FiringMode=FiringMode, Nstep=Nstep, ParInit=[PhaseInit+120 FreqInit], Ts=Ts}
      mask prompts: FiringMode "Firing Mode (1=Synchronized, 2=Continuous)"; Nstep "Total delay (in number of time step)"; ParInit "Initial phase and frequency of input: [ Phase (degree)  Freq (Hz) ]"; Ts "Sample time:"
      mask init:
      | PhaseInit=ParInit(1);
      | FreqInit=ParInit(2);
  Mux{,1..3} (4 alike) : Mux  Inputs=6
  V->pu : Gain  Gain=1/sqrt(3)  SaturateOnIntegerOverflow=on  OutDataTypeStr=Inherit: Same as input  ParamDataTypeStr=Inherit: Same as input
  TCR_Pulses : Outport
  TSC1_Pulses : Outport  Port=2
  TSC2_Pulses : Outport  Port=3
  TSC3_Pulses : Outport  Port=4
  wires:
  V->pu/1 -> Demux/1
  Alpha/1 -> Firing Unit AB/2(Alpha), Firing Unit BC/2(Alpha), Firing Unit CA/2(Alpha)
  TSC1_On/1 -> Firing Unit BC/3(TSC1_On), Firing Unit AB/3(TSC1_On), Firing Unit CA/3(TSC1_On)
  TSC2_On/1 -> Firing Unit CA/4(TSC2_On), Firing Unit BC/4(TSC2_On), Firing Unit AB/4(TSC2_On)
  Demux/1 -> Firing Unit AB/1(V)
  Demux/2 -> Firing Unit BC/1(V)
  Vabc/1 -> V->pu/1
  Demux/3 -> Firing Unit CA/1(V)
  Firing Unit AB/1(TCR +) -> Mux/1
  Firing Unit AB/2(TCR -) -> Mux/2
  Firing Unit BC/3(TSC1 +) -> Mux1/3
  Firing Unit BC/4(TSC1 -) -> Mux1/4
  Firing Unit BC/1(TCR +) -> Mux/3
  Firing Unit BC/2(TCR -) -> Mux/4
  Firing Unit CA/1(TCR +) -> Mux/5
  Firing Unit CA/2(TCR -) -> Mux/6
  Mux/1 -> TCR_Pulses/1
  Firing Unit AB/3(TSC1 +) -> Mux1/1
  Firing Unit AB/4(TSC1 -) -> Mux1/2
  Firing Unit CA/3(TSC1 +) -> Mux1/5
  Firing Unit CA/4(TSC1 -) -> Mux1/6
  Mux1/1 -> TSC1_Pulses/1
  Firing Unit AB/5(TSC2 +) -> Mux2/1
  Firing Unit AB/6(TSC2 -) -> Mux2/2
  Mux2/1 -> TSC2_Pulses/1
  Firing Unit BC/5(TSC2 +) -> Mux2/3
  Firing Unit BC/6(TSC2 -) -> Mux2/4
  Firing Unit CA/5(TSC2 +) -> Mux2/5
  Firing Unit CA/6(TSC2 -) -> Mux2/6
  TSC3_On/1 -> Firing Unit CA/5(TSC3_On), Firing Unit BC/5(TSC3_On), Firing Unit AB/5(TSC3_On)
  Mux3/1 -> TSC3_Pulses/1
  Firing Unit AB/7(TSC3 +) -> Mux3/1
  Firing Unit AB/8(TSC3 -) -> Mux3/2
  Firing Unit BC/7(TSC3 +) -> Mux3/3
  Firing Unit BC/8(TSC3 -) -> Mux3/4
  Firing Unit CA/7(TSC3 +) -> Mux3/5
  Firing Unit CA/8(TSC3 -) -> Mux3/6

== system MATLABPSB_BASED_MODELING_AND_Sim/SS1/SVC Controller/Measurement System ==
  Vabc : Inport  PortDimensions=3
  3-phase PLL : powerlib_extras/Discrete  Control Blocks/Discrete 3-phase PLL  Fmin=45  Par_Init=[Phase_Init Freq_Init]  ParK=[60 1400]  Ts=Ts  AGC=off
  PLL-Driven Positive-Sequence Fundamental Value : powerlib_extras/Discrete Measurements/Discrete 3-phase PLL-Driven Positive-Sequence Fundamental Value  Finit=Freq_Init  Fmin=45  Par_Init=[Mag_Init 0]  Ts=Ts
  Terminator : Terminator
  Terminator1 : Terminator
  Vmes : Outport
  wires:
  3-phase PLL/1 -> PLL-Driven Positive-Sequence Fundamental Value/1
  Vabc/1 -> PLL-Driven Positive-Sequence Fundamental Value/3, 3-phase PLL/1
  PLL-Driven Positive-Sequence Fundamental Value/2 -> Terminator1/1
  PLL-Driven Positive-Sequence Fundamental Value/1 -> Vmes/1
  3-phase PLL/2 -> Terminator/1
  3-phase PLL/3 -> PLL-Driven Positive-Sequence Fundamental Value/2

== system MATLABPSB_BASED_MODELING_AND_Sim/SS1/SVC Controller/Voltage Regulator ==
  note: Xs -> Slope in pu/100MVA
      |  Ki -> Integral gain (puB/puV/s)
  note: where:
  note: Closed-loop time constant --> Tc = [ Xs / ( Xr + Xs ) ] * To
  note: Open-loop time constant --> To = 1 / ( Ki * Xs )
  Vmes : Inport  PortDimensions=1
  Bref : Inport  Port=2  PortDimensions=1
  Vref : Inport  Port=3
  Constant : Constant  Value=OpMode
  Constant10 : Constant
  Droop : Gain  Gain=Xs  SaturateOnIntegerOverflow=on  OutDataTypeStr=Inherit: Same as input  ParamDataTypeStr=Inherit: Same as input
  Gain1 : Gain  Gain=Kp  SaturateOnIntegerOverflow=on  OutDataTypeStr=Inherit: Same as input  ParamDataTypeStr=Inherit: Same as input
  Gain2 : Gain  Gain=Ki  SaturateOnIntegerOverflow=on  OutDataTypeStr=Inherit: Same as input  ParamDataTypeStr=Inherit: Same as input
  Integrateur : DiscreteIntegrator  SampleTime=Ts  LimitOutput=on  UpperSaturationLimit=Bmax  LowerSaturationLimit=Bmin  ICPrevOutput=DiscIntNeverNeededParam  ICPrevScaledInput=DiscIntNeverNeededParam
  Prod. : Product  SaturateOnIntegerOverflow=on  InputSameDT=on  OutDataTypeStr=Inherit: Same as first input
  Relational Operator2 : RelationalOperator  Operator=~=  InputSameDT=on
  Som : Sum  Inputs=-+  SaturateOnIntegerOverflow=on  InputSameDT=on  OutDataTypeStr=Inherit: Same as first input
  Som1 : Sum  Inputs=-+  SaturateOnIntegerOverflow=on  InputSameDT=on  OutDataTypeStr=Inherit: Same as first input
  Som2 : Sum  SaturateOnIntegerOverflow=on  InputSameDT=on  OutDataTypeStr=Inherit: Same as first input
  Switch2 : Switch  Threshold=0.5  SaturateOnIntegerOverflow=on  InputSameDT=on
  Unit Delay1 : UnitDelay  SampleTime=Ts
  Bsvc : Outport  InitialOutput=0
  wires:
  Constant/1 -> Relational Operator2/2
  Som1/1 -> Gain2/1, Gain1/1  "err"
  Gain2/1 -> Integrateur/1
  Relational Operator2/1 -> Switch2/2
  Bref/1 -> Switch2/1
  Som2/1 -> Switch2/3
  Switch2/1 -> Unit Delay1/1, Bsvc/1
  Vmes/1 -> Prod./1, Som/1
  Vref/1 -> Som/2
  Droop/1 -> Som1/1
  Som/1 -> Som1/2
  Constant10/1 -> Relational Operator2/1
  Unit Delay1/1 -> Prod./2
  Integrateur/1 -> Som2/2
  Gain1/1 -> Som2/1
  Prod./1 -> Droop/1

== system MATLABPSB_BASED_MODELING_AND_Sim/SS1/TSC1/Subsystem ==
  In1 : Inport
  AC Voltage Source : powerlib/Electrical Sources/AC Voltage Source  Amplitude=25e3*sqrt(2)  Phase=0  Frequency=50  SampleTime=0  Measurements=None
  Ground1 : powerlib/Elements/Ground  LConnTagsString=a
  ThAB- : powerlib/Power Electronics/Thyristor  Ron=Ron  Lon=Lon  Vf=Vf  IC=IC  Rs=Rs  Cs=Cs  Measurements=off
      settings: AttributesFormatString=\n
  a : PMIOPort  Tag=PMCPort  Port=1  Side=Left
  k : PMIOPort  Tag=PMCPort  Port=2  Side=Right
  wires:
  In1/1 -> ThAB-/1
  connections:
  ThAB-/LConn1 -- a/RConn1
  Ground1/LConn1 -- AC Voltage Source/LConn1
  AC Voltage Source/RConn1 -- k/RConn1 -- ThAB-/RConn1

== system MATLABPSB_BASED_MODELING_AND_Sim/SS2/SVC Controller/3-phase signal generator ==
  Constant : Constant  Value=[0 -2*pi/3 2*pi/3]-2*pi/180
  Gain : Gain  Gain=2*pi*60  SaturateOnIntegerOverflow=on  OutDataTypeStr=Inherit: Same as input  ParamDataTypeStr=Inherit: Same as input
  Gain1 : Gain  Gain=0.9998  SaturateOnIntegerOverflow=on  OutDataTypeStr=Inherit: Same as input  ParamDataTypeStr=Inherit: Same as input
  Sum : Sum  Inputs=|++  SaturateOnIntegerOverflow=on
  Trigonometric Function : Trigonometry
  t : DigitalClock  SampleTime=Ts
  abc : Outport
  wires:
  Constant/1 -> Sum/2
  Sum/1 -> Trigonometric Function/1
  Trigonometric Function/1 -> Gain1/1
  t/1 -> Gain/1
  Gain/1 -> Sum/1
  Gain1/1 -> abc/1

== system MATLABPSB_BASED_MODELING_AND_Sim/SS2/SVC Controller/Distribution Unit ==
  note: Bsec = ( 2 - Alpha/90 + sin(2*Alpha)/PI ) * Bsec_nom
  Bsvc : Inport  PortDimensions=1
  Bprim-->Bsec : Fcn  Expr=u[1]/(1 + u[1]*Xf_xfo*100e6/Pnom_xfo)
  Bsec --> Alpha : Lookup  InputValues=B  Table=A  SaturateOnIntegerOverflow=on
  Saturation : Saturate  UpperLimit=0  LowerLimit=Bpu_TCR
  Sum1 : Sum  Inputs=+---  SaturateOnIntegerOverflow=on  InputSameDT=on  OutDataTypeStr=Inherit: Same as first input
  TSC1 : Relay  OnSwitchValue=0  OffSwitchValue=-1 * hyst_svc
  TSC1+TSC2 : Relay  OnSwitchValue=0+ Bpu_TSC  OffSwitchValue=-1 * hyst_svc + Bpu_TSC
  TSC1+TSC2+TSC3 : Relay  OnSwitchValue=0+ 2*Bpu_TSC  OffSwitchValue=-1 * hyst_svc + 2*Bpu_TSC
  pu100_puLnom : Gain  Gain=-1/Bpu_TCR  SaturateOnIntegerOverflow=on  OutDataTypeStr=Inherit: Same as input  ParamDataTypeStr=Inherit: Same as input
  pu100_puLnom1 : Gain  Gain=Bpu_TSC  SaturateOnIntegerOverflow=on  OutDataTypeStr=Inherit: Same as input  ParamDataTypeStr=Inherit: Same as input
  pu100_puLnom2 : Gain  Gain=Bpu_TSC  SaturateOnIntegerOverflow=on  OutDataTypeStr=Inherit: Same as input  ParamDataTypeStr=Inherit: Same as input
  pu100_puLnom3 : Gain  Gain=Bpu_TSC  SaturateOnIntegerOverflow=on  OutDataTypeStr=Inherit: Same as input  ParamDataTypeStr=Inherit: Same as input
  Alpha : Outport  InitialOutput=0
  TSC1_On : Outport  Port=2  InitialOutput=0
  TSC2_On : Outport  Port=3  InitialOutput=0
  TSC3_On : Outport  Port=4  InitialOutput=0
  wires:
  pu100_puLnom/1 -> Bsec --> Alpha/1
  Bsec --> Alpha/1 -> Alpha/1
  Bsvc/1 -> Bprim-->Bsec/1
  Bprim-->Bsec/1 -> TSC1/1, TSC1+TSC2/1, TSC1+TSC2+TSC3/1, Sum1/1
  Saturation/1 -> pu100_puLnom/1
  Sum1/1 -> Saturation/1
  pu100_puLnom2/1 -> Sum1/3
  pu100_puLnom3/1 -> Sum1/2
  TSC1/1 -> pu100_puLnom3/1, TSC1_On/1
  TSC1+TSC2/1 -> pu100_puLnom2/1, TSC2_On/1
  pu100_puLnom1/1 -> Sum1/4
  TSC1+TSC2+TSC3/1 -> pu100_puLnom1/1, TSC3_On/1

== system MATLABPSB_BASED_MODELING_AND_Sim/SS2/SVC Controller/Firing Unit ==
  Vabc : Inport  PortDimensions=3
  Alpha : Inport  Port=2  PortDimensions=1
  TSC1_On : Inport  Port=3  PortDimensions=1
  TSC2_On : Inport  Port=4  PortDimensions=1
  TSC3_On : Inport  Port=5  PortDimensions=1
  Demux : Demux  Outputs=3
  Firing Unit AB : Subsystem  mask{FiringMode=FiringMode, Nstep=Nstep, ParInit=[PhaseInit FreqInit], Ts=Ts}
      mask prompts: FiringMode "Firing Mode (1=Synchronized, 2=Continuous)"; Nstep "Total delay (in number of time step)"; ParInit "Initial phase and frequency of input: [ Phase (degree)  Freq (Hz) ]"; Ts "Sample time:"
      mask init:
      | PhaseInit=ParInit(1);
      | FreqInit=ParInit(2);
  Firing Unit BC : Subsystem  mask{FiringMode=FiringMode, Nstep=Nstep, ParInit=[PhaseInit-120 FreqInit], Ts=Ts}
      mask prompts: FiringMode "Firing Mode (1=Synchronized, 2=Continuous)"; Nstep "Total delay (in number of time step)"; ParInit "Initial phase and frequency of input: [ Phase (degree)  Freq (Hz) ]"; Ts "Sample time:"
      mask init:
      | PhaseInit=ParInit(1);
      | FreqInit=ParInit(2);
  Firing Unit CA : Subsystem  mask{FiringMode=FiringMode, Nstep=Nstep, ParInit=[PhaseInit+120 FreqInit], Ts=Ts}
      mask prompts: FiringMode "Firing Mode (1=Synchronized, 2=Continuous)"; Nstep "Total delay (in number of time step)"; ParInit "Initial phase and frequency of input: [ Phase (degree)  Freq (Hz) ]"; Ts "Sample time:"
      mask init:
      | PhaseInit=ParInit(1);
      | FreqInit=ParInit(2);
  Mux{,1..3} (4 alike) : Mux  Inputs=6
  V->pu : Gain  Gain=1/sqrt(3)  SaturateOnIntegerOverflow=on  OutDataTypeStr=Inherit: Same as input  ParamDataTypeStr=Inherit: Same as input
  TCR_Pulses : Outport
  TSC1_Pulses : Outport  Port=2
  TSC2_Pulses : Outport  Port=3
  TSC3_Pulses : Outport  Port=4
  wires:
  V->pu/1 -> Demux/1
  Alpha/1 -> Firing Unit AB/2(Alpha), Firing Unit BC/2(Alpha), Firing Unit CA/2(Alpha)
  TSC1_On/1 -> Firing Unit BC/3(TSC1_On), Firing Unit AB/3(TSC1_On), Firing Unit CA/3(TSC1_On)
  TSC2_On/1 -> Firing Unit CA/4(TSC2_On), Firing Unit BC/4(TSC2_On), Firing Unit AB/4(TSC2_On)
  Demux/1 -> Firing Unit AB/1(V)
  Demux/2 -> Firing Unit BC/1(V)
  Vabc/1 -> V->pu/1
  Demux/3 -> Firing Unit CA/1(V)
  Firing Unit AB/1(TCR +) -> Mux/1
  Firing Unit AB/2(TCR -) -> Mux/2
  Firing Unit BC/3(TSC1 +) -> Mux1/3
  Firing Unit BC/4(TSC1 -) -> Mux1/4
  Firing Unit BC/1(TCR +) -> Mux/3
  Firing Unit BC/2(TCR -) -> Mux/4
  Firing Unit CA/1(TCR +) -> Mux/5
  Firing Unit CA/2(TCR -) -> Mux/6
  Mux/1 -> TCR_Pulses/1
  Firing Unit AB/3(TSC1 +) -> Mux1/1
  Firing Unit AB/4(TSC1 -) -> Mux1/2
  Firing Unit CA/3(TSC1 +) -> Mux1/5
  Firing Unit CA/4(TSC1 -) -> Mux1/6
  Mux1/1 -> TSC1_Pulses/1
  Firing Unit AB/5(TSC2 +) -> Mux2/1
  Firing Unit AB/6(TSC2 -) -> Mux2/2
  Mux2/1 -> TSC2_Pulses/1
  Firing Unit BC/5(TSC2 +) -> Mux2/3
  Firing Unit BC/6(TSC2 -) -> Mux2/4
  Firing Unit CA/5(TSC2 +) -> Mux2/5
  Firing Unit CA/6(TSC2 -) -> Mux2/6
  TSC3_On/1 -> Firing Unit CA/5(TSC3_On), Firing Unit BC/5(TSC3_On), Firing Unit AB/5(TSC3_On)
  Mux3/1 -> TSC3_Pulses/1
  Firing Unit AB/7(TSC3 +) -> Mux3/1
  Firing Unit AB/8(TSC3 -) -> Mux3/2
  Firing Unit BC/7(TSC3 +) -> Mux3/3
  Firing Unit BC/8(TSC3 -) -> Mux3/4
  Firing Unit CA/7(TSC3 +) -> Mux3/5
  Firing Unit CA/8(TSC3 -) -> Mux3/6

== system MATLABPSB_BASED_MODELING_AND_Sim/SS2/SVC Controller/Measurement System ==
  Vabc : Inport  PortDimensions=3
  3-phase PLL : powerlib_extras/Discrete  Control Blocks/Discrete 3-phase PLL  Fmin=45  Par_Init=[Phase_Init Freq_Init]  ParK=[60 1400]  Ts=Ts  AGC=off
  PLL-Driven Positive-Sequence Fundamental Value : powerlib_extras/Discrete Measurements/Discrete 3-phase PLL-Driven Positive-Sequence Fundamental Value  Finit=Freq_Init  Fmin=45  Par_Init=[Mag_Init 0]  Ts=Ts
  Terminator : Terminator
  Terminator1 : Terminator
  Vmes : Outport
  wires:
  3-phase PLL/1 -> PLL-Driven Positive-Sequence Fundamental Value/1
  Vabc/1 -> PLL-Driven Positive-Sequence Fundamental Value/3, 3-phase PLL/1
  PLL-Driven Positive-Sequence Fundamental Value/2 -> Terminator1/1
  PLL-Driven Positive-Sequence Fundamental Value/1 -> Vmes/1
  3-phase PLL/2 -> Terminator/1
  3-phase PLL/3 -> PLL-Driven Positive-Sequence Fundamental Value/2

== system MATLABPSB_BASED_MODELING_AND_Sim/SS2/SVC Controller/Voltage Regulator ==
  note: Xs -> Slope in pu/100MVA
      |  Ki -> Integral gain (puB/puV/s)
  note: where:
  note: Closed-loop time constant --> Tc = [ Xs / ( Xr + Xs ) ] * To
  note: Open-loop time constant --> To = 1 / ( Ki * Xs )
  Vmes : Inport  PortDimensions=1
  Bref : Inport  Port=2  PortDimensions=1
  Vref : Inport  Port=3
  Constant : Constant  Value=OpMode
  Constant10 : Constant
  Droop : Gain  Gain=Xs  SaturateOnIntegerOverflow=on  OutDataTypeStr=Inherit: Same as input  ParamDataTypeStr=Inherit: Same as input
  Gain1 : Gain  Gain=Kp  SaturateOnIntegerOverflow=on  OutDataTypeStr=Inherit: Same as input  ParamDataTypeStr=Inherit: Same as input
  Gain2 : Gain  Gain=Ki  SaturateOnIntegerOverflow=on  OutDataTypeStr=Inherit: Same as input  ParamDataTypeStr=Inherit: Same as input
  Integrateur : DiscreteIntegrator  SampleTime=Ts  LimitOutput=on  UpperSaturationLimit=Bmax  LowerSaturationLimit=Bmin  ICPrevOutput=DiscIntNeverNeededParam  ICPrevScaledInput=DiscIntNeverNeededParam
  Prod. : Product  SaturateOnIntegerOverflow=on  InputSameDT=on  OutDataTypeStr=Inherit: Same as first input
  Relational Operator2 : RelationalOperator  Operator=~=  InputSameDT=on
  Som : Sum  Inputs=-+  SaturateOnIntegerOverflow=on  InputSameDT=on  OutDataTypeStr=Inherit: Same as first input
  Som1 : Sum  Inputs=-+  SaturateOnIntegerOverflow=on  InputSameDT=on  OutDataTypeStr=Inherit: Same as first input
  Som2 : Sum  SaturateOnIntegerOverflow=on  InputSameDT=on  OutDataTypeStr=Inherit: Same as first input
  Switch2 : Switch  Threshold=0.5  SaturateOnIntegerOverflow=on  InputSameDT=on
  Unit Delay1 : UnitDelay  SampleTime=Ts
  Bsvc : Outport  InitialOutput=0
  wires:
  Constant/1 -> Relational Operator2/2
  Som1/1 -> Gain2/1, Gain1/1  "err"
  Gain2/1 -> Integrateur/1
  Relational Operator2/1 -> Switch2/2
  Bref/1 -> Switch2/1
  Som2/1 -> Switch2/3
  Switch2/1 -> Unit Delay1/1, Bsvc/1
  Vmes/1 -> Prod./1, Som/1
  Vref/1 -> Som/2
  Droop/1 -> Som1/1
  Som/1 -> Som1/2
  Constant10/1 -> Relational Operator2/1
  Unit Delay1/1 -> Prod./2
  Integrateur/1 -> Som2/2
  Gain1/1 -> Som2/1
  Prod./1 -> Droop/1

== system MATLABPSB_BASED_MODELING_AND_Sim/SS2/TSC1/Subsystem ==
  In1 : Inport
  AC Voltage Source : powerlib/Electrical Sources/AC Voltage Source  Amplitude=15e3*sqrt(2)  Phase=120  Frequency=50  SampleTime=0  Measurements=None
  Ground1 : powerlib/Elements/Ground  LConnTagsString=a
  ThAB- : powerlib/Power Electronics/Thyristor  Ron=Ron  Lon=Lon  Vf=Vf  IC=IC  Rs=Rs  Cs=Cs  Measurements=off
      settings: AttributesFormatString=\n
  a : PMIOPort  Tag=PMCPort  Port=1  Side=Left
  k : PMIOPort  Tag=PMCPort  Port=2  Side=Right
  wires:
  In1/1 -> ThAB-/1
  connections:
  ThAB-/LConn1 -- a/RConn1
  Ground1/LConn1 -- AC Voltage Source/LConn1
  AC Voltage Source/RConn1 -- k/RConn1 -- ThAB-/RConn1
